simulink model "basemodel"  (R2021a)
settings: Solver=VariableStepAuto  StartTime=0.0  StopTime=0.09  RelTol=1e-3
libraries: spsVoltageMeasurementLib x7, spsSeriesRLCBranchLib x6, spsCurrentMeasurementLib x5, spsIGBTDiodeLib x3, spsMeanPhasorLib x3, spsDiodeLib x2, spsDCVoltageSourceLib x1, spspowerguiLib x1
settings Model: Creator=Dell  LastModifiedBy=Dell

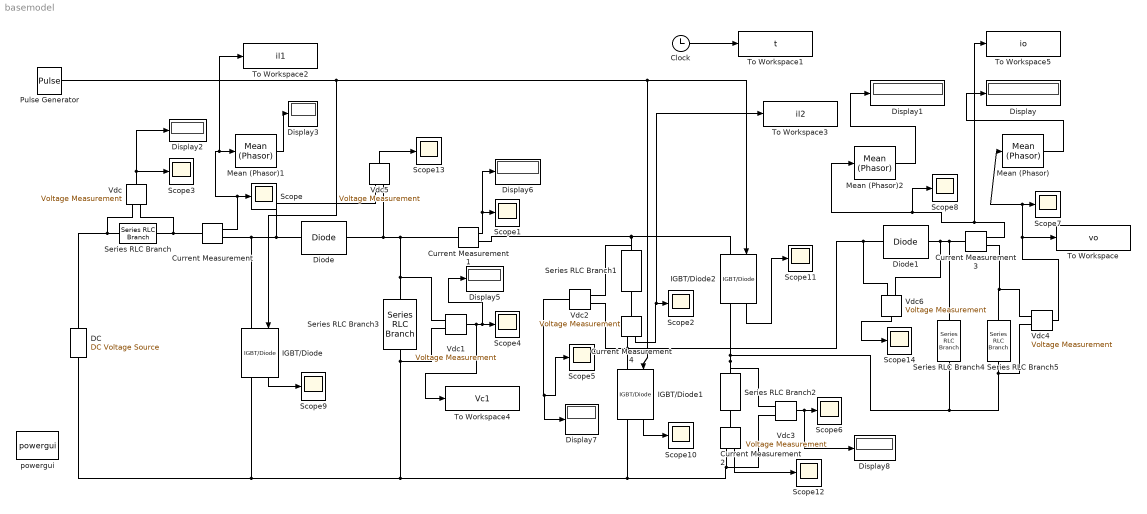
== system basemodel ==
  Clock : Clock
  Current Measurement{,1..4} (5 alike) : spsCurrentMeasurementLib/Current Measurement  PhasorSimulation=off  OutputType=Complex  PSBequivalent=0
  "DC " : spsDCVoltageSourceLib/DC Voltage Source  Amplitude=20  Measurements=Voltage
  Diode : spsDiodeLib/Diode  Ron=0.01  Lon=0  Vf=0.3  IC=0  UseSnubber=off  Rs=50000  Cs=250e-9  Measurements=off
  Diode1 : spsDiodeLib/Diode  Ron=0.01  Lon=0  Vf=0.3  IC=0  UseSnubber=off  Rs=50000  Cs=250e-9  Measurements=off
  Display{,1..3,5..8} (8 alike) : Display
  IGBT/Diode : spsIGBTDiodeLib/IGBT//Diode  Ron=1e-3  Rs=1e5  Cs=inf  Measurements=on
  IGBT/Diode1 : spsIGBTDiodeLib/IGBT//Diode  Ron=1e-3  Rs=1e5  Cs=inf  Measurements=on
  IGBT/Diode2 : spsIGBTDiodeLib/IGBT//Diode  Ron=1e-3  Rs=1e5  Cs=inf  Measurements=on
  Mean (Phasor) : spsMeanPhasorLib/Mean (Phasor)  Freq=50  Vinit=0  Ts=0
      settings: SourceProductBaseCode=PS
  Mean (Phasor)1 : spsMeanPhasorLib/Mean (Phasor)  Freq=50  Vinit=0  Ts=0
      settings: SourceProductBaseCode=PS
  Mean (Phasor)2 : spsMeanPhasorLib/Mean (Phasor)  Freq=50  Vinit=0  Ts=0
      settings: SourceProductBaseCode=PS
  Pulse Generator : DiscretePulseGenerator  PulseType=Time based  Period=1/60000  PulseWidth=70
  Scope{,1..14} (15 alike) : Scope
  Series RLC Branch : spsSeriesRLCBranchLib/Series RLC Branch  LConnTagsString=__new0  RConnTagsString=__new0  BranchType=L  Resistance=1  Inductance=11.33e-6  SetiL0=off  InitialCurrent=0  Capacitance=1e-6  Setx0=off  InitialVoltage=0  Measurements=None
  Series RLC Branch1 : spsSeriesRLCBranchLib/Series RLC Branch  LConnTagsString=__new0  RConnTagsString=__new0  BranchType=L  Resistance=1  Inductance=17.17e-6  SetiL0=off  InitialCurrent=0  Capacitance=1e-6  Setx0=off  InitialVoltage=0  Measurements=None
  Series RLC Branch2 : spsSeriesRLCBranchLib/Series RLC Branch  LConnTagsString=__new0  RConnTagsString=__new0  BranchType=L  Resistance=1  Inductance=17.17e-6  SetiL0=off  InitialCurrent=0  Capacitance=1e-6  Setx0=off  InitialVoltage=0  Measurements=None
  Series RLC Branch3 : spsSeriesRLCBranchLib/Series RLC Branch  LConnTagsString=__new0  RConnTagsString=__new0  BranchType=C  Resistance=1  Inductance=1e-3  SetiL0=off  InitialCurrent=0  Capacitance=20.81e-6  Setx0=off  InitialVoltage=0  Measurements=None
  Series RLC Branch4 : spsSeriesRLCBranchLib/Series RLC Branch  LConnTagsString=__new0  RConnTagsString=__new0  BranchType=C  Resistance=1  Inductance=1e-3  SetiL0=off  InitialCurrent=0  Capacitance=500e-6  Setx0=off  InitialVoltage=0  Measurements=None
  Series RLC Branch5 : spsSeriesRLCBranchLib/Series RLC Branch  LConnTagsString=__new0  RConnTagsString=__new0  BranchType=R  Resistance=1.44  Inductance=1e-3  SetiL0=off  InitialCurrent=0  Capacitance=1e-6  Setx0=off  InitialVoltage=0  Measurements=None
  To Workspace : ToWorkspace  VariableName=vo  SampleTime=-1
  To Workspace1 : ToWorkspace  VariableName=t  SampleTime=-1
  To Workspace2 : ToWorkspace  VariableName=il1  SampleTime=-1
  To Workspace3 : ToWorkspace  VariableName=il2  SampleTime=-1
  To Workspace4 : ToWorkspace  VariableName=Vc1  SampleTime=-1
  To Workspace5 : ToWorkspace  VariableName=io  SampleTime=-1
  Vdc{,1..6} (7 alike) : spsVoltageMeasurementLib/Voltage Measurement  PhasorSimulation=off  OutputType=Complex  PSBequivalent=0
  powergui : spspowerguiLib/powergui  Priority=1  SimulationMode=Continuous  SampleTime=1e-5  frequency=60  Iterations=50  frequencyindice=0  Pbase=100e6  ErrMax=1e-4  UnitsV=kV  UnitsW=MW  buscounter=0  FunctionMessages=off  echomessages=off  EnableUseOfTLC=off  CurrentSourceSwitches=off  DisableSnubberDevices=off  DisableRonSwitches=off  DisableVfSwitches=off  DisplayEquations=off  AutomaticDiscreteSolvers=off  SolverType=Tustin/Backward Euler (TBE)  Interpol=off  ExternalGateDelay=off  methode=off  Ts=100  x0status=blocks  SPID=on  SwTol=0  HookPort=off  NonlinearTolerance=1e-4  nMaxIteration=100  ContinueOnMaxIteration=off  RestoreLinks=warning  ResistiveCurrentMeasurement=off  Frange=[0:2:500]  Ylog=off  Xlog=on  ShowGrid=off  save=off  variable=ZData  structure=0  ZoomFFT=off  StartTime=0.0  cycles=1  DisplayStyle=1  fundamental=60  FreqAxis=off  MaxFrequency=1000  frequencyindicesteady=1  RmsSteady=1  display=off
  wires:
  Current Measurement/1 -> To Workspace2/1, Mean (Phasor)1/1, Scope/1
  Current Measurement1/1 -> Display6/1, Scope1/1
  Vdc/1 -> Scope3/1, Display2/1
  Vdc1/1 -> To Workspace4/1, Display5/1, Scope4/1
  Vdc2/1 -> Display7/1, Scope5/1
  Vdc3/1 -> Display8/1, Scope6/1
  Vdc4/1 -> To Workspace/1, Mean (Phasor)/1, Scope7/1
  Pulse Generator/1 -> IGBT/Diode/1, IGBT/Diode1/1, IGBT/Diode2/1
  Current Measurement3/1 -> To Workspace5/1, Scope8/1, Mean (Phasor)2/1
  IGBT/Diode2/1 -> Scope11/1
  IGBT/Diode1/1 -> Scope10/1
  Mean (Phasor)/1 -> Display/1
  Mean (Phasor)1/1 -> Display3/1
  Mean (Phasor)2/1 -> Display1/1
  Current Measurement4/1 -> To Workspace3/1, Scope2/1
  Current Measurement2/1 -> Scope12/1
  IGBT/Diode/1 -> Scope9/1
  Vdc5/1 -> Scope13/1
  Vdc6/1 -> Scope14/1
  Clock/1 -> To Workspace1/1
  connections:
  Current Measurement/LConn1 -- Vdc/LConn2 -- Series RLC Branch/RConn1
  Diode/LConn1 -- Current Measurement/RConn1 -- IGBT/Diode/LConn1 -- Vdc5/LConn1
  "DC "/RConn1 -- Vdc/LConn1 -- Series RLC Branch/LConn1
  Current Measurement1/LConn1 -- Vdc1/LConn1 -- Series RLC Branch3/LConn1 -- Diode/RConn1 -- Vdc5/LConn2
  Current Measurement1/RConn1 -- Vdc2/LConn1 -- Series RLC Branch1/LConn1 -- IGBT/Diode2/LConn1
  Vdc2/LConn2 -- Current Measurement4/RConn1 -- IGBT/Diode1/LConn1 -- Vdc6/LConn1 -- Diode1/LConn1
  "DC "/LConn1 -- IGBT/Diode/RConn1 -- Vdc1/LConn2 -- Series RLC Branch3/RConn1 -- Vdc3/LConn2 -- Current Measurement2/RConn1 -- IGBT/Diode1/RConn1
  Diode1/RConn1 -- Vdc6/LConn2 -- Current Measurement3/LConn1 -- Series RLC Branch4/LConn1
  Vdc4/LConn1 -- Current Measurement3/RConn1 -- Series RLC Branch5/LConn1
  Current Measurement2/LConn1 -- Series RLC Branch2/RConn1
  Vdc3/LConn1 -- Series RLC Branch4/RConn1 -- Vdc4/LConn2 -- Series RLC Branch5/RConn1 -- IGBT/Diode2/RConn1 -- Series RLC Branch2/LConn1
  Current Measurement4/LConn1 -- Series RLC Branch1/RConn1
